simulink model "lab6_3"  (R2018b)
settings: Solver=VariableStepAuto  StartTime=0.0  StopTime=10.0  RelTol=1e-3
settings Model: Creator=mllax8  LastModifiedBy=mllax8

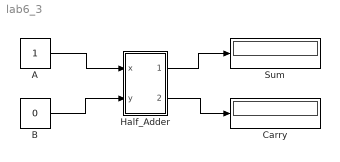
== system lab6_3 ==
  A : Constant  OutDataTypeStr=boolean
  B : Constant  Value=0  OutDataTypeStr=boolean
  Carry : Display
  Half_Adder : Subsystem
  Sum : Display
  wires:
  A/1 -> Half_Adder/1(x)
  Half_Adder/1(Sum) -> Sum/1
  B/1 -> Half_Adder/2(y)
  Half_Adder/2(Carry) -> Carry/1

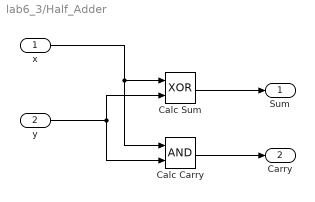
== system lab6_3/Half_Adder ==
  x : Inport
  y : Inport  Port=2
  Calc Carry : Logic  AllPortsSameDT=off  OutDataTypeStr=boolean
  Calc Sum : Logic  Operator=XOR  AllPortsSameDT=off  OutDataTypeStr=boolean
  Sum : Outport
  Carry : Outport  Port=2
  wires:
  Calc Carry/1 -> Carry/1
  x/1 -> Calc Carry/1, Calc Sum/1
  Calc Sum/1 -> Sum/1
  y/1 -> Calc Sum/2, Calc Carry/2
